simulink model "tank_based_force_pos"  (R2020b)
settings: Solver=ode45  StartTime=0.0  StopTime=10  FixedStep=Ts  MinStep=1e-5  RelTol=1e-5
undefined symbols (not defined in the file): A, Be, beta, Bh_i, Bm, Bs, delayT, Dh, Dm, Ds, Fc, Fip, Hd, Hm_init, Hs_init, Jh_i, Ke, Kh, Kh_i, Km, Ks, Mm, Ms, tlcAlpha, Ts, xe
libraries: simulink x2, cstblocks x1
settings Model: Creator=simon  LastModifiedBy=SimoneCremasco
settings SolverCC: AlgebraicLoopSolver=LineSearch

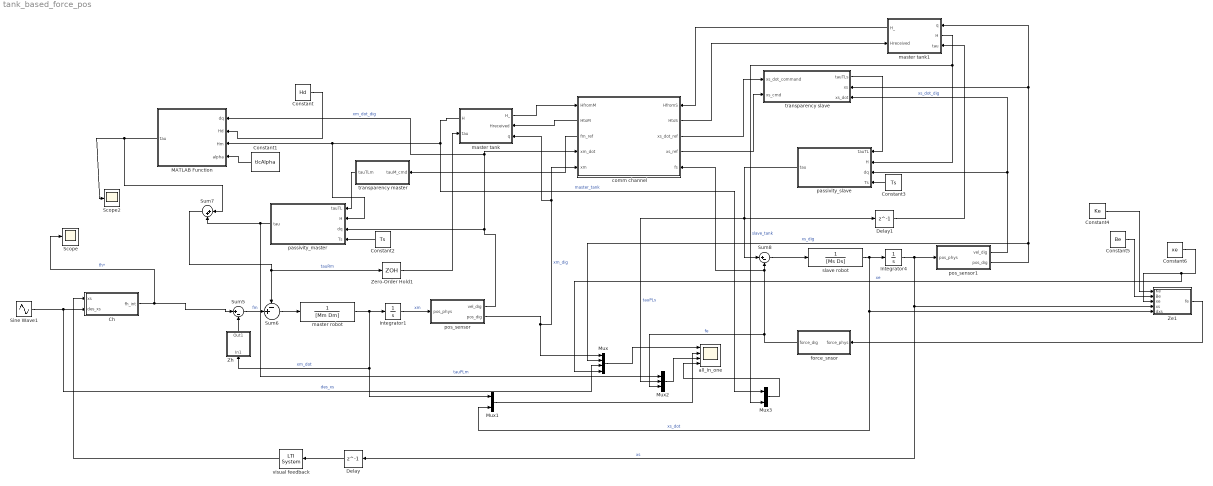
== system tank_based_force_pos ==
  Ch : Subsystem
  Constant : Constant  Value=Hd
  Constant1 : Constant  Value=tlcAlpha
  Constant2 : Constant  Value=Ts
  Constant3 : Constant  Value=Ts
  Constant4 : Constant  Value=Ke
  Constant5 : Constant  Value=Be
  Constant6 : Constant  Value=xe
  Delay : Delay  DelayLength=1  SampleTime=Ts
  Delay1 : Delay  DelayLength=1  SampleTime=Ts
  Integrator1 : Integrator
  Integrator4 : Integrator
  MATLAB Function : MATLAB Function  TreatAsAtomicUnit=on
  Mux : Mux
  Mux1 : Mux  Inputs=2
  Mux2 : Mux  Inputs=3
  Mux3 : Mux  Inputs=2
  Scope : Scope
  Scope2 : Scope
  Sine Wave1 : Sin  Amplitude=A  Frequency=2*pi*Fc  SampleTime=0
  Sum5 : Sum  Inputs=|+-
  Sum6 : Sum  Inputs=-+|
  Sum7 : Sum  Inputs=|++
  Sum8 : Sum  Inputs=|+-
  Ze1 : MATLAB Function  TreatAsAtomicUnit=on
  Zero-Order Hold1 : ZeroOrderHold  SampleTime=Ts
  Zh : Subsystem
  all_in_one : Scope  NumInputPorts=4
  comm channel : Subsystem
      settings: PortSchema="{\"entries\":[{\"content\":{\"sides\":[{\"content\":{\"connectorIds\":[\"In1\",\"Out3\",\"Out4\",\"Out5\",\"In2\"]},\"type\":\"ConnectorPlacement.EquallySpacedRectSide\",\"uuid\":\"1c070cf8-9aa7-4f7b-8e2f-2632c2893f69\"},{\"content\":{\"connectorIds\":[\"In3\",\"Out1\",\"Out2\",\"In4\",\"In5\"],\"side\":\"RIGHT\"},\"type\":\"ConnectorPlacement.EquallySpacedRectSide\",\"uuid\":\"32173565-3523-4dfc-9820-763c87098354\"},{\"content\":{\"connectorIds\":[],\"side\":\"TOP\"},\"type\":\"ConnectorPlacement.EquallySpacedRectSide\",\"uuid\":\"13187df6-bf6f-436e-a2ee-34150977e6a8\"},{\"content\":{\"connectorIds\":[],\"side\":\"HIDDEN\"},\"type\":\"ConnectorPlacement.EquallySpacedRectSide\",\"uuid\":\"1e5bcdd7-6028-40f7-b524-727817e519ff\"}]},\"type\":\"ConnectorPlacement.EquallySpacedConnector\",\"uuid\":\"c84d0440-83b9-4b92-a10a-1f72bb115b54\"}],\"packageUris\":[\"http://schema.mathworks.com/mf0/Connector/R2020b\"],\"version\":\"1.0\"}"
  force_snsor : Subsystem
  master robot : TransferFcn  Denominator=[Mm Dm]
  master tank : Subsystem
      settings: PortSchema="{\"entries\":[{\"content\":{\"sides\":[{\"content\":{\"connectorIds\":[\"Out2\",\"In1\",\"In2\"]},\"type\":\"ConnectorPlacement.EquallySpacedRectSide\",\"uuid\":\"482b0a11-f044-49fa-a74d-4dac8b5b787b\"},{\"content\":{\"connectorIds\":[\"Out1\",\"In3\"],\"side\":\"RIGHT\"},\"type\":\"ConnectorPlacement.EquallySpacedRectSide\",\"uuid\":\"b0c369ed-ae40-43d8-b393-bca9f7720d62\"},{\"content\":{\"connectorIds\":[],\"side\":\"TOP\"},\"type\":\"ConnectorPlacement.EquallySpacedRectSide\",\"uuid\":\"ff021616-d6aa-4c0a-874b-a9ebe947c92c\"},{\"content\":{\"connectorIds\":[],\"side\":\"BOTTOM\"},\"type\":\"ConnectorPlacement.EquallySpacedRectSide\",\"uuid\":\"4e18ee96-bca7-41b6-9abb-5b593b41c296\"},{\"content\":{\"connectorIds\":[],\"side\":\"HIDDEN\"},\"type\":\"ConnectorPlacement.EquallySpacedRectSide\",\"uuid\":\"be815b34-35c7-4c6f-8c8b-4a812b3d12e9\"}]},\"type\":\"ConnectorPlacement.EquallySpacedConnector\",\"uuid\":\"78552b8a-5f1c-4815-a807-de98f58b7f2e\"}],\"packageUris\":[\"http://schema.mathworks.com/mf0/Connector/R2020b\"],\"version\":\"1.0\"}"
  master tank1 : Subsystem
      settings: PortSchema="{\"entries\":[{\"content\":{\"sides\":[{\"content\":{\"connectorIds\":[\"In1\",\"Out2\",\"In2\"]},\"type\":\"ConnectorPlacement.EquallySpacedRectSide\",\"uuid\":\"482b0a11-f044-49fa-a74d-4dac8b5b787b\"},{\"content\":{\"connectorIds\":[\"Out1\",\"In3\"],\"side\":\"RIGHT\"},\"type\":\"ConnectorPlacement.EquallySpacedRectSide\",\"uuid\":\"b0c369ed-ae40-43d8-b393-bca9f7720d62\"},{\"content\":{\"connectorIds\":[],\"side\":\"TOP\"},\"type\":\"ConnectorPlacement.EquallySpacedRectSide\",\"uuid\":\"ff021616-d6aa-4c0a-874b-a9ebe947c92c\"},{\"content\":{\"connectorIds\":[],\"side\":\"BOTTOM\"},\"type\":\"ConnectorPlacement.EquallySpacedRectSide\",\"uuid\":\"4e18ee96-bca7-41b6-9abb-5b593b41c296\"},{\"content\":{\"connectorIds\":[],\"side\":\"HIDDEN\"},\"type\":\"ConnectorPlacement.EquallySpacedRectSide\",\"uuid\":\"be815b34-35c7-4c6f-8c8b-4a812b3d12e9\"}]},\"type\":\"ConnectorPlacement.EquallySpacedConnector\",\"uuid\":\"78552b8a-5f1c-4815-a807-de98f58b7f2e\"}],\"packageUris\":[\"http://schema.mathworks.com/mf0/Connector/R2020b\"],\"version\":\"1.0\"}"
  passivity_master : MATLAB Function  TreatAsAtomicUnit=on
  passivity_slave : MATLAB Function  TreatAsAtomicUnit=on
  pos_sensor : Subsystem
  pos_sensor1 : Subsystem
  slave robot : TransferFcn  Denominator=[Ms Ds]
  transparency master : Subsystem
  transparency slave : Subsystem
      settings: PortSchema="{\"entries\":[{\"content\":{\"sides\":[{\"content\":{\"connectorIds\":[\"In1\",\"In2\"]},\"type\":\"ConnectorPlacement.EquallySpacedRectSide\",\"uuid\":\"c8f256d1-8287-4bc6-9264-40c0684f6acd\"},{\"content\":{\"connectorIds\":[\"Out1\",\"In3\",\"In4\"],\"side\":\"RIGHT\"},\"type\":\"ConnectorPlacement.EquallySpacedRectSide\",\"uuid\":\"cb9f571e-93fc-426e-a4f2-aa96ae3bd6b3\"},{\"content\":{\"connectorIds\":[],\"side\":\"TOP\"},\"type\":\"ConnectorPlacement.EquallySpacedRectSide\",\"uuid\":\"b9b91304-f20e-4a66-aa64-b99c686ee85a\"},{\"content\":{\"connectorIds\":[],\"side\":\"HIDDEN\"},\"type\":\"ConnectorPlacement.EquallySpacedRectSide\",\"uuid\":\"c3abcf5a-e3b9-4b9a-a4b1-68c5725be1f4\"}]},\"type\":\"ConnectorPlacement.EquallySpacedConnector\",\"uuid\":\"83907002-acbd-4948-aeba-a43201e13c19\"}],\"packageUris\":[\"http://schema.mathworks.com/mf0/Connector/R2020b\"],\"version\":\"1.0\"}"
  visual feedback : cstblocks/LTI System  sys=1  IC=[]
  wires:
  Zh/1(Out1) -> Sum5/2
  Integrator1/1 -> pos_sensor/1(pos_phys)  "xm"
  master robot/1 -> Integrator1/1, Mux1/1, Zh/1(In1)  "xm_dot"
  Ch/1(fh_int) -> Scope/1, Sum5/1  "fh*"
  Sum6/1 -> master robot/1
  pos_sensor/2(pos_dig) -> Mux/1, master tank/2(q), comm channel/5(xm)  "xm_dig"
  Sum5/1 -> Sum6/2  "fm"
  Sum7/1 -> Sum6/1, Zero-Order Hold1/1  "tauRm"
  pos_sensor/1(vel_dig) -> MATLAB Function/1(dq), comm channel/4(xm_dot), passivity_master/3(dq)  "xm_dot_dig"
  slave robot/1 -> Mux1/2, Ze1/5(dxs), Integrator4/1  "xs_dot"
  Integrator4/1 -> Delay/1, Ze1/4(xs), pos_sensor1/1(pos_phys)  "xs"
  pos_sensor1/2(pos_dig) -> Mux/2, master tank1/1(q), transparency slave/3(xs)  "xs_dig"
  pos_sensor1/1(vel_dig) -> transparency slave/4(xs_dot), passivity_slave/3(dq)  "xs_dot_dig"
  Sum8/1 -> slave robot/1
  Constant4/1 -> Ze1/1(Ke)
  Constant5/1 -> Ze1/2(Be)
  Constant6/1 -> Mux/4, Ze1/3(xe)  "xe"
  Ze1/1(fe) -> force_snsor/1(force_phys)
  master tank/1(H) -> Mux3/1, passivity_master/2(H), MATLAB Function/3(Hm)  "master_tank"
  comm channel/1(HtoM) -> master tank/1(Hreceived)
  transparency master/1(tauTLm) -> passivity_master/1(tauTL)
  transparency slave/1(tauTLs) -> passivity_slave/1(tauTL)
  comm channel/3(HtoS) -> master tank1/3(Hreceived)
  Constant/1 -> MATLAB Function/2(Hd)
  comm channel/4(xs_dot_ref) -> transparency slave/1(xs_dot_command)
  comm channel/2(fm_ref) -> transparency master/1(tauM_cmd)
  Zero-Order Hold1/1 -> master tank/3(tau)
  Sine Wave1/1 -> Mux/3, Ch/2(des_xs)  "des_xs"
  visual feedback/1 -> Ch/1(xs)
  Delay/1 -> visual feedback/1
  comm channel/5(xs_ref) -> transparency slave/2(xs_cmd)
  master tank/2(H_) -> comm channel/3(HfromM)
  master tank1/1(H_) -> comm channel/1(HfromS)
  Delay1/1 -> master tank1/2(tau)
  Constant1/1 -> MATLAB Function/4(alpha)
  MATLAB Function/1(tau) -> Sum7/1, Scope2/1
  Constant2/1 -> passivity_master/4(Ts)
  Constant3/1 -> passivity_slave/4(Ts)
  master tank1/2(H) -> Mux3/2, passivity_slave/2(H)  "slave_tank"
  force_snsor/1(force_dig) -> Mux2/3, comm channel/2(fs), Sum8/2  "fe"
  passivity_master/1(tau) -> Sum7/2, Mux2/1  "tauPLm"
  passivity_slave/1(tau) -> Sum8/1, Delay1/1, Mux2/2  "tauPLs"
  Mux/1 -> all_in_one/1
  Mux1/1 -> all_in_one/2
  Mux2/1 -> all_in_one/3
  Mux3/1 -> all_in_one/4

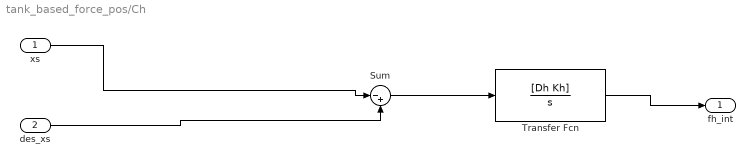
== system tank_based_force_pos/Ch ==
  xs : Inport
  des_xs : Inport  Port=2
  Sum : Sum  Inputs=|-+
  Transfer Fcn : TransferFcn  Numerator=[Dh Kh]  Denominator=[1 0]
  fh_int : Outport
  wires:
  xs/1 -> Sum/1
  des_xs/1 -> Sum/2
  Sum/1 -> Transfer Fcn/1
  Transfer Fcn/1 -> fh_int/1

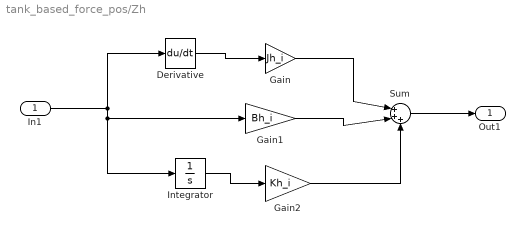
== system tank_based_force_pos/Zh ==
  In1 : Inport
  Derivative : Derivative
  Gain : Gain  Gain=Jh_i
  Gain1 : Gain  Gain=Bh_i
  Gain2 : Gain  Gain=Kh_i
  Integrator : Integrator
  Sum : Sum  Inputs=|+++
  Out1 : Outport
  wires:
  Derivative/1 -> Gain/1
  Integrator/1 -> Gain2/1
  In1/1 -> Integrator/1, Gain1/1, Derivative/1
  Gain/1 -> Sum/1
  Gain1/1 -> Sum/2
  Gain2/1 -> Sum/3
  Sum/1 -> Out1/1

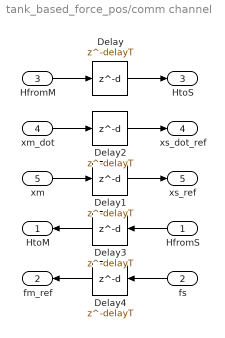
== system tank_based_force_pos/comm channel ==
  HfromS : Inport
  fs : Inport  Port=2
  HfromM : Inport  Port=3
  xm_dot : Inport  Port=4
  xm : Inport  Port=5
  Delay{,1..4} (5 alike) : Delay  DelayLength=delayT  SampleTime=Ts
  HtoM : Outport
  fm_ref : Outport  Port=2
  HtoS : Outport  Port=3
  xs_dot_ref : Outport  Port=4
  xs_ref : Outport  Port=5
  wires:
  HfromS/1 -> Delay3/1
  xm_dot/1 -> Delay2/1
  fs/1 -> Delay4/1
  Delay4/1 -> fm_ref/1
  xm/1 -> Delay1/1
  Delay1/1 -> xs_ref/1
  Delay2/1 -> xs_dot_ref/1
  HfromM/1 -> Delay/1
  Delay/1 -> HtoS/1
  Delay3/1 -> HtoM/1

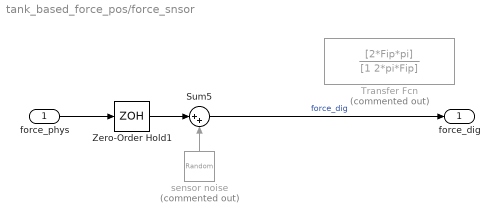
== system tank_based_force_pos/force_snsor ==
  force_phys : Inport
  Sum5 : Sum  Inputs=|++
  Transfer Fcn : TransferFcn  Commented=on  Numerator=[2*Fip*pi]  Denominator=[1 2*pi*Fip]
  Zero-Order Hold1 : ZeroOrderHold  SampleTime=Ts
  sensor noise : RandomNumber  Commented=on  Variance=0.0000001  SampleTime=Ts
  force_dig : Outport
  wires:
  force_phys/1 -> Zero-Order Hold1/1
  sensor noise/1 -> Sum5/2
  Zero-Order Hold1/1 -> Sum5/1
  Sum5/1 -> force_dig/1  "force_dig"

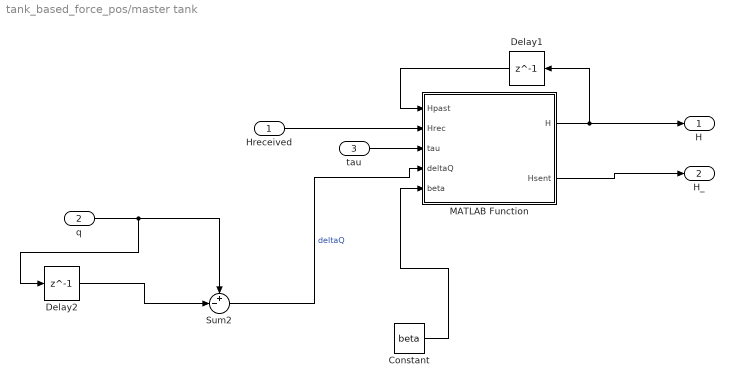
== system tank_based_force_pos/master tank ==
  Hreceived : Inport
  q : Inport  Port=2
  tau : Inport  Port=3
  Constant : Constant  Value=beta
  Delay1 : Delay  DelayLength=1  InitialCondition=Hm_init  SampleTime=Ts
  Delay2 : Delay  DelayLength=1  SampleTime=Ts
  MATLAB Function : MATLAB Function  TreatAsAtomicUnit=on
  Sum2 : Sum  Inputs=+-|
  H : Outport
  H_ : Outport  Port=2
  wires:
  Delay2/1 -> Sum2/2
  q/1 -> Delay2/1, Sum2/1
  MATLAB Function/2(Hsent) -> H_/1
  Constant/1 -> MATLAB Function/5(beta)
  Sum2/1 -> MATLAB Function/4(deltaQ)  "deltaQ"
  Hreceived/1 -> MATLAB Function/2(Hrec)
  tau/1 -> MATLAB Function/3(tau)
  MATLAB Function/1(H) -> Delay1/1, H/1
  Delay1/1 -> MATLAB Function/1(Hpast)

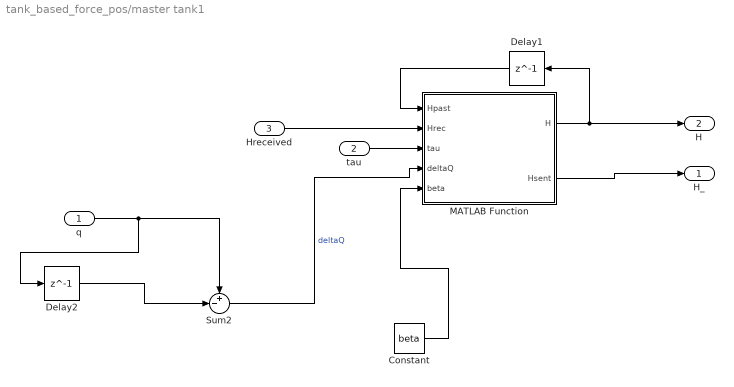
== system tank_based_force_pos/master tank1 ==
  q : Inport
  tau : Inport  Port=2
  Hreceived : Inport  Port=3
  Constant : Constant  Value=beta
  Delay1 : Delay  DelayLength=1  InitialCondition=Hs_init  SampleTime=Ts
  Delay2 : Delay  DelayLength=1  SampleTime=Ts
  MATLAB Function : MATLAB Function  TreatAsAtomicUnit=on
  Sum2 : Sum  Inputs=+-|
  H_ : Outport
  H : Outport  Port=2
  wires:
  Delay2/1 -> Sum2/2
  q/1 -> Delay2/1, Sum2/1
  MATLAB Function/2(Hsent) -> H_/1
  Constant/1 -> MATLAB Function/5(beta)
  Sum2/1 -> MATLAB Function/4(deltaQ)  "deltaQ"
  Hreceived/1 -> MATLAB Function/2(Hrec)
  tau/1 -> MATLAB Function/3(tau)
  MATLAB Function/1(H) -> Delay1/1, H/1
  Delay1/1 -> MATLAB Function/1(Hpast)

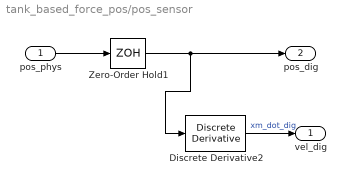
== system tank_based_force_pos/pos_sensor ==
  pos_phys : Inport
  Discrete Derivative2 : simulink/Discrete/Discrete Derivative  gainval=1.0  ICPrevScaledInput=0.0  OutMin=[]  OutMax=[]  OutDataType=fixdt(1, 16)  OutScaling=2^-10  DoSatur=off
  Zero-Order Hold1 : ZeroOrderHold  SampleTime=Ts
  vel_dig : Outport
  pos_dig : Outport  Port=2
  wires:
  Zero-Order Hold1/1 -> Discrete Derivative2/1, pos_dig/1
  pos_phys/1 -> Zero-Order Hold1/1
  Discrete Derivative2/1 -> vel_dig/1  "xm_dot_dig"

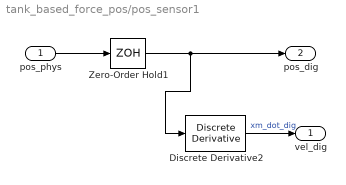
== system tank_based_force_pos/pos_sensor1 ==
  pos_phys : Inport
  Discrete Derivative2 : simulink/Discrete/Discrete Derivative  gainval=1.0  ICPrevScaledInput=0.0  OutMin=[]  OutMax=[]  OutDataType=fixdt(1, 16)  OutScaling=2^-10  DoSatur=off
  Zero-Order Hold1 : ZeroOrderHold  SampleTime=Ts
  vel_dig : Outport
  pos_dig : Outport  Port=2
  wires:
  Zero-Order Hold1/1 -> Discrete Derivative2/1, pos_dig/1
  pos_phys/1 -> Zero-Order Hold1/1
  Discrete Derivative2/1 -> vel_dig/1  "xm_dot_dig"

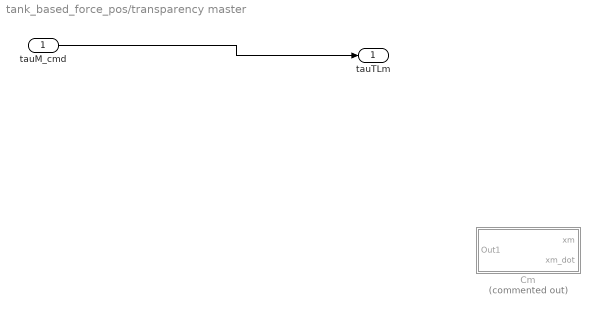
== system tank_based_force_pos/transparency master ==
  tauM_cmd : Inport
  Cm : Subsystem  Commented=on
  tauTLm : Outport
  wires:
  tauM_cmd/1 -> tauTLm/1

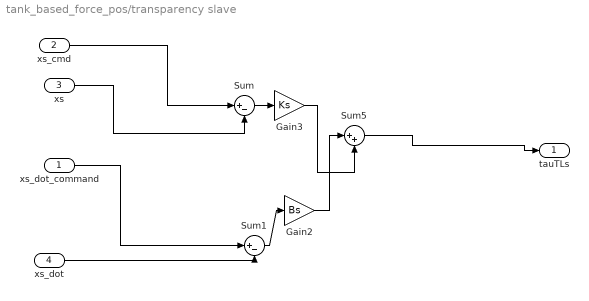
== system tank_based_force_pos/transparency slave ==
  xs_dot_command : Inport
  xs_cmd : Inport  Port=2
  xs : Inport  Port=3
  xs_dot : Inport  Port=4
  Gain2 : Gain  Gain=Bs
  Gain3 : Gain  Gain=Ks
  Sum : Sum  Inputs=|+-
  Sum1 : Sum  Inputs=|+-
  Sum5 : Sum  Inputs=|++
  tauTLs : Outport
  wires:
  Sum5/1 -> tauTLs/1
  xs/1 -> Sum/2
  xs_dot/1 -> Sum1/2
  xs_cmd/1 -> Sum/1
  xs_dot_command/1 -> Sum1/1
  Gain2/1 -> Sum5/1
  Gain3/1 -> Sum5/2
  Sum/1 -> Gain3/1
  Sum1/1 -> Gain2/1

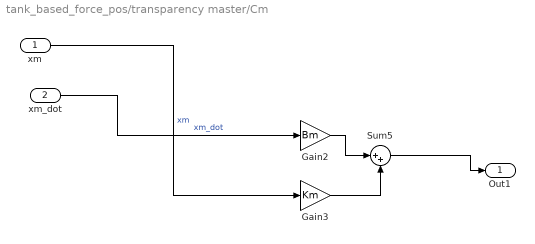
== system tank_based_force_pos/transparency master/Cm ==
  xm : Inport
  xm_dot : Inport  Port=2
  Gain2 : Gain  Gain=Bm
  Gain3 : Gain  Gain=Km
  Sum5 : Sum  Inputs=|++
  Out1 : Outport
  wires:
  xm/1 -> Gain3/1  "xm"
  Gain2/1 -> Sum5/1
  xm_dot/1 -> Gain2/1  "xm_dot"
  Gain3/1 -> Sum5/2
  Sum5/1 -> Out1/1

== matlab function tank_based_force_pos/MATLAB Function ==
  data: dq input; tau output; Hd input; Hm input; alpha input
function tau = tauTLC(dq, Hd, Hm, alpha)
if Hd <= Hm
    d = 0;
else
    d = alpha*(Hd-Hm);
end
tau = -d*dq;

== matlab function tank_based_force_pos/master tank/MATLAB Function ==
  data: Hpast input; H output; Hrec input; tau input; deltaQ input; beta input; Hsent output
function [H,Hsent] = tank(Hpast, Hrec, tau, deltaQ, beta)
Hused = tau*deltaQ;
H = Hpast+Hrec-Hused;    
Hsent = H*beta;
H = H-Hsent;

== matlab function tank_based_force_pos/master tank1/MATLAB Function ==
  data: Hpast input; H output; Hrec input; tau input; deltaQ input; beta input; Hsent output
function [H,Hsent] = tank(Hpast, Hrec, tau, deltaQ, beta)
Hused = tau*deltaQ;
H = Hpast+Hrec-Hused;    
Hsent = H*beta;
H = H-Hsent;

== matlab function tank_based_force_pos/passivity_slave ==
  data: tauTL input; H input; tau output; dq input; Ts input
function tau = tauPL(tauTL, H, dq,Ts)
if H<= 0
    tauMax1 = 0;
else
    tauMax1 = tauTL;
end
tauMax2 = H/(dq*Ts);
tau = sign(tauTL)*min([abs(tauMax1),abs(tauMax2)]);

== matlab function tank_based_force_pos/passivity_master ==
  data: tauTL input; H input; tau output; dq input; Ts input
function tau = tauPL(tauTL, H, dq,Ts)
if H<= 0
    tauMax1 = 0;
else
    tauMax1 = tauTL;
end
tauMax2 = H/(dq*Ts);
tau = sign(tauTL)*min([abs(tauMax1),abs(tauMax2)]);

== matlab function tank_based_force_pos/Ze1 ==
  data: Ke input; fe output; Be input; xe input; xs input; dxs input
function fe = env(Ke, Be, xe, xs, dxs)
    if xs > xe
        fe = Ke*(xs-xe)+Be*max(dxs, 0);
    else
        fe = 0;
    end
